simulink model "PWM"  (R2022b)
settings: Solver=VariableStepAuto  StartTime=0.0  StopTime=10.0  RelTol=1e-3
libraries: eePwmGenerator x1
settings Model: Creator=aceao  LastModifiedBy=USUARIO

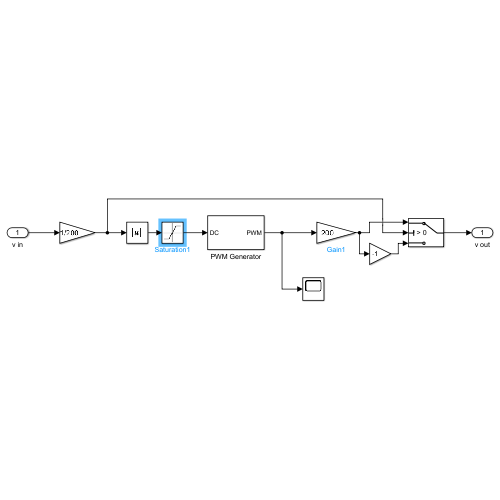
[thumbnail: Simulink's stored preview of the top-level diagram]
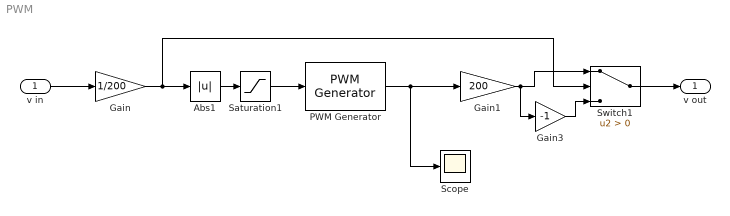
== system PWM ==
  v in : Inport
  Abs1 : Abs  SaturateOnIntegerOverflow=off
  Gain : Gain  Gain=1/200
  Gain1 : Gain  Gain=200
  Gain3 : Gain  Gain=-1
  PWM Generator : eePwmGenerator/PWM Generator  CarrCount=Up  Tper=1/3e4  Tdelay=0  Ts=0
  Saturation1 : Saturate  UpperLimit=1  LowerLimit=0
  Scope : Scope
  Switch1 : Switch  Criteria=u2 > Threshold  SaturateOnIntegerOverflow=off  InputSameDT=off
  v out : Outport
  wires:
  v in/1 -> Gain/1
  PWM Generator/1 -> Gain1/1, Scope/1
  Gain/1 -> Switch1/2, Abs1/1
  Abs1/1 -> Saturation1/1
  Saturation1/1 -> PWM Generator/1
  Gain3/1 -> Switch1/3
  Gain1/1 -> Gain3/1, Switch1/1
  Switch1/1 -> v out/1
